simulink model "led_ADC_FW"  (R2024b)
settings: Solver=ode4  StartTime=0.0  StopTime=Inf  FixedStep=Ts  RelTol=1e-3  EnableMultiTasking=on
InitFcn:
  | Ts=1e-4
model workspace (MAT data in the model file):
  encoderResolution = 2000
  hallOffset = '0.5'
  indexOffset = 850
  polePairs = '4'
libraries: c2837xDlib x5, simulink x4, c280xlib x2, c2802xlib x1
(part 1 of 2)
settings Model: ExtModeTrigDuration=8  Creator=matti  LastModifiedBy=Administrator
settings SolverCC: AlgebraicLoopSolver=TrustRegion
settings DataIOCC: LimitDataPoints=on  SaveFormat=Array  SignalLoggingSaveFormat=ModelDataLogs  SaveOutput=off  SaveTime=off  ReturnWorkspaceOutputs=off
settings OptimizationCC: DefaultUnderspecifiedDataType=single  OptimizeBlockIOStorage=off  BufferReuse=off  GlobalBufferReuse=off  ExpressionFolding=off  ExpressionDepthLimit=2147483647  LocalBlockOutputs=off  InitFltsAndDblsToZero=on  NoFixptDivByZeroProtection=on  EfficientFloat2IntCast=on  EfficientMapNaN2IntZero=off  LifeSpan=Inf  MaxStackSize=1024  OptimizeDataStoreBuffers=off  BusAssignmentInplaceUpdate=off  EfficientTunableParamExpr=on
settings DebuggingCC: ReadBeforeWriteMsg=DisableAll  WriteAfterWriteMsg=DisableAll  WriteAfterReadMsg=DisableAll  CheckSSInitialOutputMsg=off  UnderspecifiedInitializationDetection=Classic  MergeDetectMultiDrivingBlocksExec=none  SignalResolutionControl=TryResolveAllWithWarning  SolverPrmCheckMsg=warning  InheritedTsInSrcMsg=none  MultiTaskDSMMsg=none  MultiTaskCondExecSysMsg=none  TasksWithSamePriorityMsg=none  SigSpecEnsureSampleTimeMsg=none  IntegerOverflowMsg=none  ParameterPrecisionLossMsg=none  FcnCallInpInsideContextMsg=warning  UnconnectedInputMsg=warning  UnconnectedOutputMsg=warning  UnconnectedLineMsg=warning  StateNameClashWarn=warning  SFUnexpectedBacktrackingDiag=warning  SFNoUnconditionalDefaultTransitionDiag=warning  SFExecutionAtInitializationDiag=none  IntegerSaturationMsg=none  ArithmeticOperatorsInVariantConditions=warning
settings HardwareCC: ProdBitPerChar=16  ProdBitPerInt=16  ProdBitPerPointer=32  ProdBitPerSizeT=32  ProdBitPerPtrDiffT=32  ProdLargestAtomicInteger=Integer  ProdLargestAtomicFloat=None  ProdWordSize=16  ProdLongLongMode=on  ProdHWDeviceType=Texas Instruments->C2000  TargetBitPerChar=16  TargetBitPerInt=16  TargetBitPerPointer=16  TargetLargestAtomicInteger=Integer  TargetIntDivRoundTo=Zero  TargetEndianess=LittleEndian  TargetWordSize=16  TargetHWDeviceType=TI C2000  HardwareBoardFeatureSet=SoCBlockset
settings ModelReferenceCC: EnableRefExpFcnMdlSchedulingChecks=on  PropagateSignalLabelsOutOfModel=off
settings SFSimCC: SimUseLocalCustomCode=off  MATLABDynamicMemAlloc=off  CustomCodeUndefinedFunction=UseInterfaceOnly
settings RTWCC: Description=Embedded Coder  SystemTargetFile=ert.tlc  HardwareBoard=TI Delfino F28379D LaunchPad  TemplateMakefile=ert_default_tmf  GenerateReport=on  RTWUseLocalCustomCode=off  CustomHeaderCode=#include<stdlib.h>  Toolchain=Texas Instruments Code Composer Studio (C2000)  IncludeHyperlinkInReport=on  LaunchReport=on  CodeProfilingSaveOptions=MetricsOnly  GenerateTraceInfo=on  GenerateTraceReport=on  GenerateTraceReportSl=on  GenerateTraceReportSf=on  GenerateTraceReportEml=on  GPUComputeCapability=3.5
settings CodeAppCC: IgnoreCustomStorageClasses=off  CustomSymbolStrType=$N$R$M  StateflowObjectComments=on  InternalIdentifier=Classic
settings ERTTargetCC: CodeReplacementLibrary=TI C28x  MultiwordLength=2048  SupportContinuousTime=on  ExtModeTransport=4  ExtModeStaticAlloc=on  ExtModeAutomaticAllocSize=off  ExtModeStaticAllocSize=10000  ExtModeMexFile=ext_xcp  ExtModeIntrfLevel=Level2 - Open  InlinedParameterPlacement=Hierarchical  ConvertIfToSwitch=off  SuppressUnreachableDefaultCases=off  MemSecPackage=tic2000demospkg  MemSecFuncExecute=code_ramfuncs  DynamicArrayContainerType=coder::array
settings ConfigComp: CovMetricSettings=dw  CovSaveCumulativeToWorkspaceVar=on  CovSaveSingleToWorkspaceVar=on  CovExternalEMLEnable=off  CovSFcnEnable=off
settings SimscapeCC: SimscapeNormalizeSystem=off

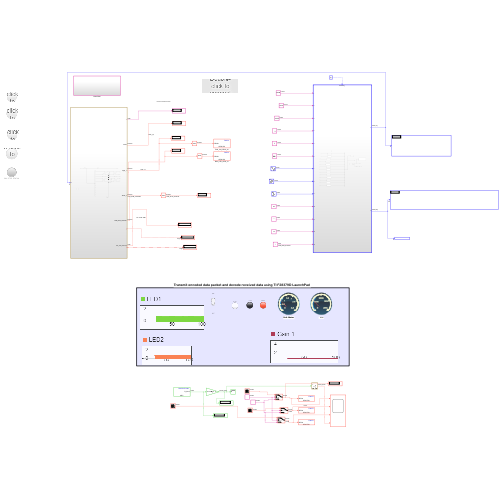
[thumbnail: Simulink's stored preview of the top-level diagram]
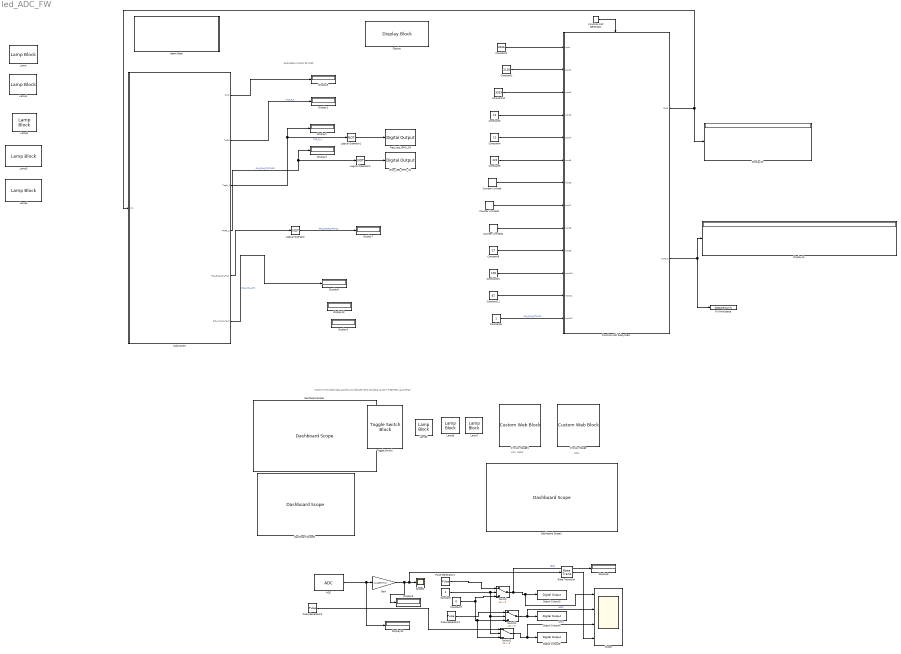
== system led_ADC_FW ==
  note: SHAILESH KUMAR SR MGR
  note: Votl- Meter
  note: Transmit encoded data packet and decode received data using TI F28379D LaunchPad
  note: RPM
  ADC : c2802xlib/ADC  blkParamProc=C2000_Type4  ADCModule=D  samplingMode=Single sample mode  ADCResolution=12-bit (Single-ended input)  useSOC1=SOC0  useSOC2=SOC0_SOC1  SOCAcquisitionWindow=15  SOCTriggerSource=Software  SOCInterruptTrigger=No ADCINT  Ts=0.001  dType=uint16  postInterrupt=off  interruptSel=ADCINT1  ADCINTContinuous=on  endma=off  chdma=1  conv1=ADCINA0  conv2=ADCINA0 and ADCINB0  conv1_Type4=ADCIN14  conv2_Type4=ADCIN0 and ADCIN1
      settings: LibrarySourceBlock=c2837xDlib/ADC
  Blue_LED_GPIO_31 : c2837xDlib/Digital Output  GPIO_Number=GPIO24~GPIO31  GPIO_Bit0=off  GPIO_BIT0_Toggle=off  GPIO_Bit1=off  GPIO_BIT1_Toggle=off  GPIO_Bit2=off  GPIO_BIT2_Toggle=off  GPIO_Bit3=off  GPIO_BIT3_Toggle=off  GPIO_Bit4=off  GPIO_BIT4_Toggle=off  GPIO_Bit5=off  GPIO_BIT5_Toggle=off  GPIO_Bit6=off  GPIO_BIT6_Toggle=off  GPIO_Bit7=on  GPIO_BIT7_Toggle=off
  Circular Gauge : CustomWebBlock  LabelPosition=Hide  ShowInitialText=on  Configuration="{\"components\":[{\"name\":\"CircularScaleComponent\",\"settings\":{\"bounds\":{\"max\":4096,\"min\":0,\"tickInterval\":\"auto\"},\"direction\":\"cw\",\"flipLimits\":0,\"innerRadius\":0.75,\"internalTickHeightScaleFactor\":1,\"labelColor\":[255,255,200],\"labelFont\":{\"font\":\"Arial\",\"fontSize\":12},\"labelRadius\":0.528,\"labelTransparency\":1,\"minorTickHeightScaleFactor\":0.2,\"needleImage\":{\"size\":[200,50],\"src\":\"data:image\\/svg+xml;base64,PD94bWwgdmVyc2lvbj0iMS4wIiBlbmNvZGluZz0idXRmLTgiPz4KPCEtLSBHZW5lcmF0b3I6IEFkb2JlIElsbHVzdHJhdG9yIDI0LjEuMiwgU1ZHIEV4cG9ydCBQbHVnLUluIC4gU1ZHIFZlcnNpb246IDYuMDAgQnVpbGQgMCkgIC0tPgo8c3ZnIHZlcnNpb249IjEuMSIgaWQ9IkxheWVyXzEiIHhtbG5zPSJodHRwOi8vd3d3LnczLm9yZy8yMDAwL3N2ZyIgeG1sbnM6eGxpbms9Imh0dHA6Ly93d3cudzMub3JnLzE5OTkveGxpbmsiIHg9IjBweCIgeT0iMHB4IgoJIHZpZXdCb3g9IjAgMCAyMDAgNTAiIHN0eWxlPSJlbmFibGUtYmFja2dyb3VuZDpuZXcgMCAwIDIwMCA1MDsiIHhtbDpzcGFjZT0icHJlc2VydmUiPgo8c3R5bGUgdHlwZT0idGV4dC9jc3MiPgoJLnN0MHtmaWxsOiNFQzIxMjc7fQo8L3N0eWxlPgo8cGF0aCBjbGFzcz0ic3QwIiBkPSJNMTYyLjgsMTMuN0MxNjksNC40LDE4MS43LDEuOSwxOTEsOC4xczExLjgsMTguOSw1LjYsMjguMnMtMTguOSwxMS44LTI4LjIsNS42bDAsMAoJQzE1OS4xLDM1LjYsMTU2LjYsMjMsMTYyLjgsMTMuN0wxNjIuOCwxMy43eiBNMTY1LjgsMTUuOGMtNS4xLDcuNi0zLjEsMTcuOSw0LjYsMjNjNy42LDUuMSwxNy45LDMuMSwyMy00LjYKCWM1LjEtNy42LDMuMS0xNy45LTQuNi0yM2wwLDBDMTgxLjIsNi4yLDE3MC45LDguMiwxNjUuOCwxNS44eiIvPgo8cGF0aCBjbGFzcz0ic3QwIiBkPSJNMC40LDI1Ljl2LTMuM2wxNTktMi41Yy0wLjcsMi42LTAuNyw1LjIsMCw3LjhMMC40LDI1Ljl6Ii8+CjxjaXJjbGUgY2xhc3M9InN0MCIgY3g9IjE3OS42IiBjeT0iMjQiIHI9IjAuNyIvPgo8L3N2Zz4K\"},\"needleOffset\":[0.18464878250906522,0],\"needleOrientation\":-45,\"needleRotation\":180,\"needleSize\":{\"height\":0.11741692305346914,\"width\":0.46108337545091255},\"outerRadius\":0.9,\"position\":[0.05,0.05,0.9,0.9],\"referencePoint\":\"auto\",\"scaleAngle\":270,\"scaleAngleOffset\":135,\"scaleColors\":[],\"scaleColorsSize\":0.2,\"scaleDirection\":\"CW\",\"scalePosition\":[0,0,1,1],\"showLabels\":1,\"showMinorTicks\":1,\"showSpanLine\":1,\"showTicks\":1,\"tickColor\":[252,252,197],\"tickTransparency\":1,\"valueBarColor\":[0,114,189],\"valueBarPosition\":[0,0,1,1],\"valueBarSize\":0.2,\"valueBarTransparency\":1}},{\"name\":\"BackgroundImageComponent\",\"settings\":{\"image\":{\"size\":[500,500],\"src\":\"data:image\\/svg+xml;base64,PD94bWwgdmVyc2lvbj0iMS4wIiBlbmNvZGluZz0iVVRGLTgiIHN0YW5kYWxvbmU9Im5vIj8+CjxzdmcKICAgeG1sbnM6ZGM9Imh0dHA6Ly9wdXJsLm9yZy9kYy9lbGVtZW50cy8xLjEvIgogICB4bWxuczpjYz0iaHR0cDovL2NyZWF0aXZlY29tbW9ucy5vcmcvbnMjIgogICB4bWxuczpyZGY9Imh0dHA6Ly93d3cudzMub3JnLzE5OTkvMDIvMjItcmRmLXN5bnRheC1ucyMiCiAgIHhtbG5zOnN2Zz0iaHR0cDovL3d3dy53My5vcmcvMjAwMC9zdmciCiAgIHhtbG5zPSJodHRwOi8vd3d3LnczLm9yZy8yMDAwL3N2ZyIKICAgeG1sbnM6 ...(+9964 chars)\"},\"position\":[0,0,1,1],\"scaleMode\":\"0\"}},{\"name\":\"ForegroundImageComponent\",\"settings\":{\"image\":{\"size\":[0,0],\"src\":\"default\",\"srcOrientation\":[]},\"isForeground\":1,\"position\":[0,0,1,1],\"scaleMode\":\"0\"}}],\"settings\":{\"BindingType\":\"signal\",\"aspectRatio\":1.032258064516129,\"backgroundColor\":[0,0,0,\"1\"],\"backgroundOffset\":1,\"backgroundOpacity\":1,\"direction\":\"cw\",\"fixedAspectRatio\":\"on\",\"flipLimits\":0,\"orientation\":\"horizontal\",\"showBackgroundColor\":false,\"value\":0,\"version\":\"R2023a\"},\"type\":\"CircularGauge\"}"
  Circular Gauge1 : CustomWebBlock  LabelPosition=Hide  ShowInitialText=on  Configuration="{\"components\":[{\"name\":\"CircularScaleComponent\",\"settings\":{\"bounds\":{\"max\":3.3,\"min\":0,\"tickInterval\":\"auto\"},\"direction\":\"cw\",\"flipLimits\":0,\"innerRadius\":0.75,\"internalTickHeightScaleFactor\":1,\"labelColor\":[255,255,200],\"labelFont\":{\"font\":\"Arial\",\"fontSize\":12},\"labelRadius\":0.528,\"labelTransparency\":1,\"minorTickHeightScaleFactor\":0.2,\"needleImage\":{\"size\":[200,50],\"src\":\"data:image\\/svg+xml;base64,PD94bWwgdmVyc2lvbj0iMS4wIiBlbmNvZGluZz0idXRmLTgiPz4KPCEtLSBHZW5lcmF0b3I6IEFkb2JlIElsbHVzdHJhdG9yIDI0LjEuMiwgU1ZHIEV4cG9ydCBQbHVnLUluIC4gU1ZHIFZlcnNpb246IDYuMDAgQnVpbGQgMCkgIC0tPgo8c3ZnIHZlcnNpb249IjEuMSIgaWQ9IkxheWVyXzEiIHhtbG5zPSJodHRwOi8vd3d3LnczLm9yZy8yMDAwL3N2ZyIgeG1sbnM6eGxpbms9Imh0dHA6Ly93d3cudzMub3JnLzE5OTkveGxpbmsiIHg9IjBweCIgeT0iMHB4IgoJIHZpZXdCb3g9IjAgMCAyMDAgNTAiIHN0eWxlPSJlbmFibGUtYmFja2dyb3VuZDpuZXcgMCAwIDIwMCA1MDsiIHhtbDpzcGFjZT0icHJlc2VydmUiPgo8c3R5bGUgdHlwZT0idGV4dC9jc3MiPgoJLnN0MHtmaWxsOiNFQzIxMjc7fQo8L3N0eWxlPgo8cGF0aCBjbGFzcz0ic3QwIiBkPSJNMTYyLjgsMTMuN0MxNjksNC40LDE4MS43LDEuOSwxOTEsOC4xczExLjgsMTguOSw1LjYsMjguMnMtMTguOSwxMS44LTI4LjIsNS42bDAsMAoJQzE1OS4xLDM1LjYsMTU2LjYsMjMsMTYyLjgsMTMuN0wxNjIuOCwxMy43eiBNMTY1LjgsMTUuOGMtNS4xLDcuNi0zLjEsMTcuOSw0LjYsMjNjNy42LDUuMSwxNy45LDMuMSwyMy00LjYKCWM1LjEtNy42LDMuMS0xNy45LTQuNi0yM2wwLDBDMTgxLjIsNi4yLDE3MC45LDguMiwxNjUuOCwxNS44eiIvPgo8cGF0aCBjbGFzcz0ic3QwIiBkPSJNMC40LDI1Ljl2LTMuM2wxNTktMi41Yy0wLjcsMi42LTAuNyw1LjIsMCw3LjhMMC40LDI1Ljl6Ii8+CjxjaXJjbGUgY2xhc3M9InN0MCIgY3g9IjE3OS42IiBjeT0iMjQiIHI9IjAuNyIvPgo8L3N2Zz4K\"},\"needleOffset\":[0.18464878250906522,0],\"needleOrientation\":-45,\"needleRotation\":180,\"needleSize\":{\"height\":0.11741692305346914,\"width\":0.46108337545091255},\"outerRadius\":0.9,\"position\":[0.05,0.05,0.9,0.9],\"referencePoint\":\"auto\",\"scaleAngle\":270,\"scaleAngleOffset\":135,\"scaleColors\":[],\"scaleColorsSize\":0.2,\"scaleDirection\":\"CW\",\"scalePosition\":[0,0,1,1],\"showLabels\":1,\"showMinorTicks\":1,\"showSpanLine\":1,\"showTicks\":1,\"tickColor\":[252,252,197],\"tickTransparency\":1,\"valueBarColor\":[0,114,189],\"valueBarPosition\":[0,0,1,1],\"valueBarSize\":0.2,\"valueBarTransparency\":1}},{\"name\":\"BackgroundImageComponent\",\"settings\":{\"image\":{\"size\":[500,500],\"src\":\"data:image\\/svg+xml;base64,PD94bWwgdmVyc2lvbj0iMS4wIiBlbmNvZGluZz0iVVRGLTgiIHN0YW5kYWxvbmU9Im5vIj8+CjxzdmcKICAgeG1sbnM6ZGM9Imh0dHA6Ly9wdXJsLm9yZy9kYy9lbGVtZW50cy8xLjEvIgogICB4bWxuczpjYz0iaHR0cDovL2NyZWF0aXZlY29tbW9ucy5vcmcvbnMjIgogICB4bWxuczpyZGY9Imh0dHA6Ly93d3cudzMub3JnLzE5OTkvMDIvMjItcmRmLXN5bnRheC1ucyMiCiAgIHhtbG5zOnN2Zz0iaHR0cDovL3d3dy53My5vcmcvMjAwMC9zdmciCiAgIHhtbG5zPSJodHRwOi8vd3d3LnczLm9yZy8yMDAwL3N2ZyIKICAgeG1sbnM6 ...(+9964 chars)\"},\"position\":[0,0,1,1],\"scaleMode\":\"0\"}},{\"name\":\"ForegroundImageComponent\",\"settings\":{\"image\":{\"size\":[0,0],\"src\":\"default\",\"srcOrientation\":[]},\"isForeground\":1,\"position\":[0,0,1,1],\"scaleMode\":\"0\"}}],\"settings\":{\"BindingType\":\"signal\",\"aspectRatio\":1.032258064516129,\"backgroundColor\":[0,0,0,\"1\"],\"backgroundOffset\":1,\"backgroundOpacity\":1,\"direction\":\"cw\",\"fixedAspectRatio\":\"on\",\"flipLimits\":0,\"orientation\":\"horizontal\",\"showBackgroundColor\":false,\"value\":0,\"version\":\"R2023a\"},\"type\":\"CircularGauge\"}"
  Constant : Constant
  Constant1 : Constant  Value=2130  OutDataTypeStr=uint16
  Constant10 : Constant  Value=100  OutDataTypeStr=uint16
  Constant11 : Constant  Value=67  OutDataTypeStr=uint16
  Constant12 : Constant  Value=3333  OutDataTypeStr=uint16
  Constant2 : Constant  Value=3046  OutDataTypeStr=uint16
  Constant3 : Constant  Value=12  OutDataTypeStr=uint16
  Constant4 : Constant  Value=11  OutDataTypeStr=uint16
  Constant5 : Constant  Value=222  OutDataTypeStr=uint16
  Constant6 : Constant  OutDataTypeStr=uint8
  Constant7 : Constant  Value=0
  Constant9 : Constant  Value=27  OutDataTypeStr=uint16
  Counter Limited : simulink/Sources/Counter Limited  uplimit=999  tsamp=-1
  Counter Limited1 : simulink/Sources/Counter Limited  uplimit=999  tsamp=-1
  Counter Limited2 : simulink/Sources/Counter Limited  uplimit=999  tsamp=-1
  Dashboard Scope : DashboardScope  Ymin=-1  Ymax=2  NormalizeYAxis=on  TicksPosition=Inside
  Dashboard Scope1 : DashboardScope  Ymin=.5  Ymax=4  UpdateMode=Scroll  NormalizeYAxis=on  TicksPosition=Inside
  Dashboard Scope2 : DashboardScope  Ymin=-1  Ymax=2  UpdateMode=Scroll  NormalizeYAxis=on  TicksPosition=Inside
  Digital Output3 : c2837xDlib/Digital Output  GPIO_Number=GPIO0~GPIO7  GPIO_Bit0=on  GPIO_BIT0_Toggle=off  GPIO_Bit1=off  GPIO_BIT1_Toggle=off  GPIO_Bit2=off  GPIO_BIT2_Toggle=off  GPIO_Bit3=off  GPIO_BIT3_Toggle=off  GPIO_Bit4=off  GPIO_BIT4_Toggle=off  GPIO_Bit5=off  GPIO_BIT5_Toggle=off  GPIO_Bit6=off  GPIO_BIT6_Toggle=off  GPIO_Bit7=off  GPIO_BIT7_Toggle=off
  Digital Output4 : c2837xDlib/Digital Output  GPIO_Number=GPIO0~GPIO7  GPIO_Bit0=off  GPIO_BIT0_Toggle=off  GPIO_Bit1=on  GPIO_BIT1_Toggle=off  GPIO_Bit2=off  GPIO_BIT2_Toggle=off  GPIO_Bit3=off  GPIO_BIT3_Toggle=off  GPIO_Bit4=off  GPIO_BIT4_Toggle=off  GPIO_Bit5=off  GPIO_BIT5_Toggle=off  GPIO_Bit6=off  GPIO_BIT6_Toggle=off  GPIO_Bit7=off  GPIO_BIT7_Toggle=off
  Digital Output5 : c2837xDlib/Digital Output  GPIO_Number=GPIO0~GPIO7  GPIO_Bit0=off  GPIO_BIT0_Toggle=off  GPIO_Bit1=off  GPIO_BIT1_Toggle=off  GPIO_Bit2=on  GPIO_BIT2_Toggle=off  GPIO_Bit3=off  GPIO_BIT3_Toggle=off  GPIO_Bit4=off  GPIO_BIT4_Toggle=off  GPIO_Bit5=off  GPIO_BIT5_Toggle=off  GPIO_Bit6=off  GPIO_BIT6_Toggle=off  GPIO_Bit7=off  GPIO_BIT7_Toggle=off
  Display : DisplayBlock  Transparency=1
  Display{1..10,13..15} (13 alike) : Display
  Function-Call Generator : simulink/Ports & Subsystems/Function-Call Generator  sample_time=0.1  numberOfIterations=1  DisallowWideOutput=off
  Function-Call Subsystem : Subsystem  TreatAsAtomicUnit=on
  Gain : Gain  Gain=(1/4095)*3.3
  Heart-Beat : Subsystem
  Lamp{,1..2,5..7} (6 alike) : LampBlock
  Lamp3 : LampBlock  LabelPosition=Bottom
  Lamp4 : LampBlock  LabelPosition=Bottom
  Logical Operator : Logic  Operator=NOT  AllPortsSameDT=off  OutDataTypeStr=boolean
  Logical Operator1 : Logic  Operator=NOT  AllPortsSameDT=off  OutDataTypeStr=boolean
  Logical Operator2 : Logic  Operator=NOT  AllPortsSameDT=off  OutDataTypeStr=boolean
  Pulse Generator1 : DiscretePulseGenerator  PulseType=Time based  Amplitude=0.5  Period=500e-3  PulseWidth=50  SampleTime=0.1
  Pulse Generator2 : DiscretePulseGenerator  PulseType=Time based  Amplitude=0.5  Period=1  PulseWidth=50  SampleTime=0.1
  Pulse Generator3 : DiscretePulseGenerator  PulseType=Time based  Amplitude=0.5  PulseWidth=50  SampleTime=0.1
  Rate Transition : RateTransition
  Red_Led_GPIO_34 : c2837xDlib/Digital Output  GPIO_Number=GPIO32~GPIO39  GPIO_Bit0=off  GPIO_BIT0_Toggle=off  GPIO_Bit1=off  GPIO_BIT1_Toggle=off  GPIO_Bit2=on  GPIO_BIT2_Toggle=off  GPIO_Bit3=off  GPIO_BIT3_Toggle=off  GPIO_Bit4=off  GPIO_BIT4_Toggle=off  GPIO_Bit5=off  GPIO_BIT5_Toggle=off  GPIO_Bit6=off  GPIO_BIT6_Toggle=off  GPIO_Bit7=off  GPIO_BIT7_Toggle=off
  Scope : Scope  NumInputPorts=4
  Scope1 : Scope
  Subsystem : Subsystem
  Switch : Switch  Criteria=u2 > Threshold  SaturateOnIntegerOverflow=off  InputSameDT=off
  Switch1 : Switch  Criteria=u2 > Threshold  SaturateOnIntegerOverflow=off  InputSameDT=off
  Switch2 : Switch  Criteria=u2 > Threshold  SaturateOnIntegerOverflow=off  InputSameDT=off
  To Workspace : ToWorkspace  VariableName=datatransmit  SampleTime=-1
      settings: Save2DSignal=2-D array (concatenate along first dimension)
  Toggle Switch : ToggleSwitchBlock  LabelPosition=Hide
      settings: Values={{'Off', 'On'}, [0 1]}
  wires:
  Subsystem/1(Out1) -> Display5/1
  Subsystem/3(Tag9_1) -> Display2/1, Logical Operator1/1  "TAG_9_1"
  Subsystem/6(DC_Link_Current) -> Display6/1  "DC_LINK_AMP"
  Subsystem/2(TAG9) -> Display1/1  "TAG_9_0"
  Logical Operator/1 -> Display7/1  "FAN_STOP_STATUS"
  Function-Call Generator/1 -> Function-Call Subsystem/Trigger
  Function-Call Subsystem/1(Out2) -> Subsystem/1(In1), Display15/1
  Constant2/1 -> Function-Call Subsystem/1(Input)
  Constant1/1 -> Function-Call Subsystem/2(Input1)
  Constant12/1 -> Function-Call Subsystem/3(Input2)
  Constant3/1 -> Function-Call Subsystem/4(Input3)
  Constant4/1 -> Function-Call Subsystem/5(Input4)
  Constant5/1 -> Function-Call Subsystem/6(Input5)
  Counter Limited/1 -> Function-Call Subsystem/7(Input6)
  Counter Limited1/1 -> Function-Call Subsystem/8(Input7)
  Counter Limited2/1 -> Function-Call Subsystem/9(Input8)
  Constant9/1 -> Function-Call Subsystem/10(Input9)
  Constant10/1 -> Function-Call Subsystem/11(Input10)
  Constant11/1 -> Function-Call Subsystem/12(Input11)
  Constant6/1 -> Function-Call Subsystem/13(Input12)  "FAN_RUN_STATUS"
  Function-Call Subsystem/2(Output) -> To Workspace/1, Display14/1
  Logical Operator1/1 -> Red_Led_GPIO_34/1
  Logical Operator2/1 -> Blue_LED_GPIO_31/1
  Subsystem/4(TAG9_2) -> Display3/1, Logical Operator2/1  "FAN_RUN_STATUSS"
  Subsystem/5(FAN_RUN_STATUS) -> Logical Operator/1
  ? -> Display13/1
  ? -> Display4/1
  Pulse Generator3/1 -> Switch2/1
  Rate Transition/1 -> Scope/4
  Pulse Generator1/1 -> Switch/1
  Pulse Generator2/1 -> Switch1/1
  ADC/1 -> Display10/1, Gain/1
  Switch1/1 -> Scope/2, Digital Output4/1  "LED2"
  Constant/1 -> Switch2/2, Switch1/2, Switch/2
  Gain/1 -> Display9/1, Rate Transition/1, Scope1/1
  Constant7/1 -> Switch/3, Switch2/3, Switch1/3
  Switch/1 -> Display8/1, Scope/1, Digital Output3/1  "LED1"
  Switch2/1 -> Scope/3, Digital Output5/1  "LED3"

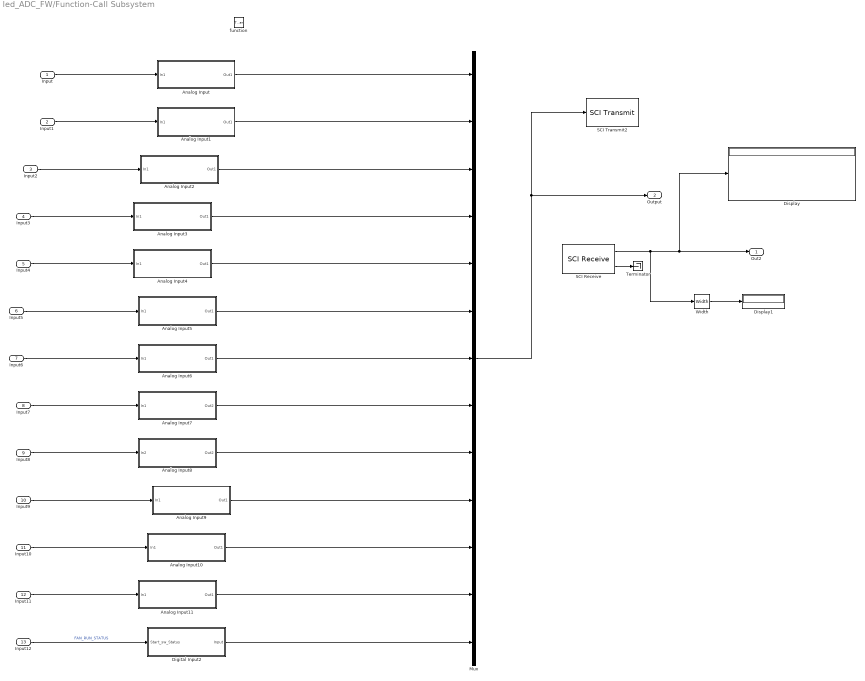
== system led_ADC_FW/Function-Call Subsystem ==
  Input : Inport
  Input1 : Inport  Port=2
  Input2 : Inport  Port=3
  Input3 : Inport  Port=4
  Input4 : Inport  Port=5
  Input5 : Inport  Port=6
  Input6 : Inport  Port=7
  Input7 : Inport  Port=8
  Input8 : Inport  Port=9
  Input9 : Inport  Port=10
  Input10 : Inport  Port=11
  Input11 : Inport  Port=12
  Input12 : Inport  Port=13
  function : TriggerPort  TriggerType=function-call  VariantControl=(inherit)
  Analog Input : Subsystem
  Analog Input1 : Subsystem
  Analog Input10 : Subsystem
  Analog Input11 : Subsystem
  Analog Input2 : Subsystem
  Analog Input3 : Subsystem
  Analog Input4 : Subsystem
  Analog Input5 : Subsystem
  Analog Input6 : Subsystem
  Analog Input7 : Subsystem
  Analog Input8 : Subsystem
  Analog Input9 : Subsystem
  Digital Input2 : Subsystem
  Display : Display
  Display1 : Display
  Mux : Mux  Inputs=13
  SCI Receive : c280xlib/SCI Receive  Priority=2  sciModule=B  dataHead='S'  headerCheckMaxCount=16  dataTail='E'  dataType=uint8  dataLenOptions=Length via dialog  dataDim=11  maxDataLength=1  initValue=0  errOption=Output the last received value  errValue=0  sampleTime=-1  blockingMode=off  timeOut=inf  outputStatus=on
      settings: LibrarySourceBlock=c2837xDlib/SCI Receive
  SCI Transmit2 : c280xlib/SCI Transmit  sciModule=B  dataHead='S'  dataTail='E'  frameSize=[1 49]  blockingMode=on  outputStatus=off
      settings: LibrarySourceBlock=c2837xDlib/SCI Transmit
  Terminator : Terminator
  Width : Width  DataType=uint8
  Out2 : Outport
  Output : Outport  Port=2
  wires:
  SCI Receive/1 -> Width/1, Display/1, Out2/1
  SCI Receive/2 -> Terminator/1
  Digital Input2/1(Input) -> Mux/13
  Analog Input/1(Out1) -> Mux/1
  Input/1 -> Analog Input/1(In1)
  Input12/1 -> Digital Input2/1(Start_sw_Status)  "FAN_RUN_STATUS"
  Mux/1 -> SCI Transmit2/1, Output/1
  Width/1 -> Display1/1
  Input1/1 -> Analog Input1/1(In1)
  Analog Input1/1(Out1) -> Mux/2
  Input2/1 -> Analog Input2/1(In1)
  Analog Input2/1(Out1) -> Mux/3
  Input3/1 -> Analog Input3/1(In1)
  Analog Input3/1(Out1) -> Mux/4
  Input4/1 -> Analog Input4/1(In1)
  Analog Input4/1(Out1) -> Mux/5
  Input5/1 -> Analog Input5/1(In1)
  Analog Input5/1(Out1) -> Mux/6
  Input6/1 -> Analog Input6/1(In1)
  Analog Input6/1(Out1) -> Mux/7
  Input7/1 -> Analog Input7/1(In1)
  Analog Input7/1(Out2) -> Mux/8
  Input8/1 -> Analog Input8/1(In2)
  Analog Input8/1(Out2) -> Mux/9
  Input9/1 -> Analog Input9/1(In1)
  Analog Input9/1(Out1) -> Mux/10
  Input10/1 -> Analog Input10/1(In1)
  Analog Input10/1(Out1) -> Mux/11
  Input11/1 -> Analog Input11/1(In1)
  Analog Input11/1(Out1) -> Mux/12

== system led_ADC_FW/Heart-Beat ==

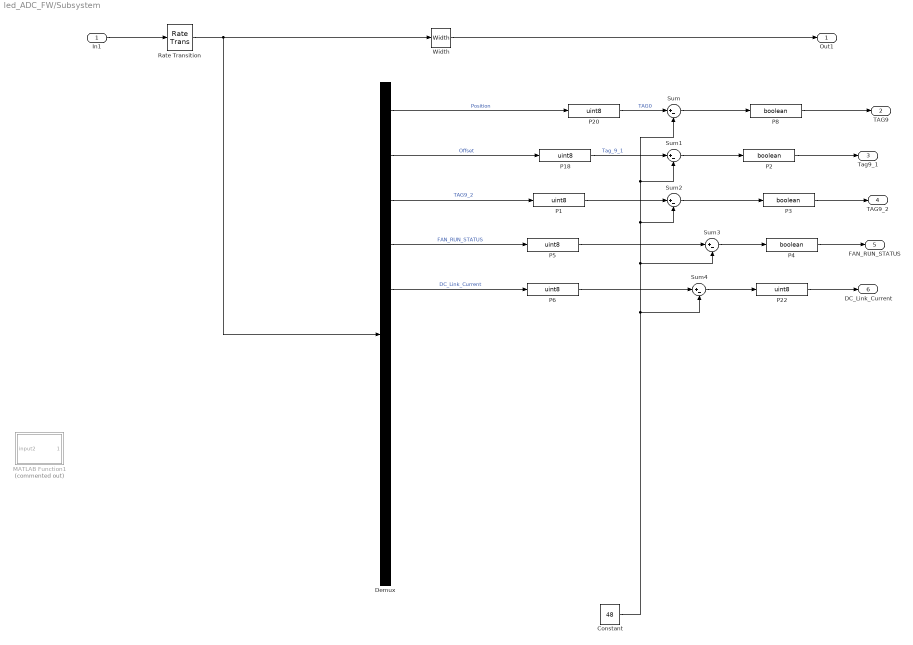
== system led_ADC_FW/Subsystem ==
  In1 : Inport
  Constant : Constant  Value=48  OutDataTypeStr=uint8
  Demux : Demux  Outputs=11
  MATLAB Function1 : MATLAB Function  Commented=on  TreatAsAtomicUnit=on
  P{1,5..6,18,20,22} (6 alike) : DataTypeConversion  OutDataTypeStr=uint8  SaturateOnIntegerOverflow=off  RndMeth=Floor
  P{2..4,8} (4 alike) : DataTypeConversion  OutDataTypeStr=boolean  SaturateOnIntegerOverflow=off  RndMeth=Floor
  Rate Transition : RateTransition
  Sum{,1..4} (5 alike) : Sum  Inputs=|+-
  Width : Width  DataType=uint8
  Out1 : Outport
  TAG9 : Outport  Port=2
  Tag9_1 : Outport  Port=3
  TAG9_2 : Outport  Port=4
  FAN_RUN_STATUS : Outport  Port=5
  DC_Link_Current : Outport  Port=6
  wires:
  Demux/1 -> P20/1  "Position"
  P1/1 -> Sum2/1
  P3/1 -> TAG9_2/1
  Sum1/1 -> P2/1
  P2/1 -> Tag9_1/1
  Sum/1 -> P8/1
  P18/1 -> Sum1/1  "Tag_9_1"
  P6/1 -> Sum4/1
  Demux/5 -> P6/1  "DC_Link_Current"
  P4/1 -> FAN_RUN_STATUS/1
  Demux/4 -> P5/1  "FAN_RUN_STATUS"
  P5/1 -> Sum3/1
  Sum3/1 -> P4/1
  Demux/3 -> P1/1  "TAG9_2"
  Sum4/1 -> P22/1
  Demux/2 -> P18/1  "Offset"
  Sum2/1 -> P3/1
  In1/1 -> Rate Transition/1
  Width/1 -> Out1/1
  P20/1 -> Sum/1  "TAG0"
  Rate Transition/1 -> Demux/1, Width/1
  P8/1 -> TAG9/1
  P22/1 -> DC_Link_Current/1
  Constant/1 -> Sum4/2, Sum3/2, Sum2/2, Sum1/2, Sum/2

== system led_ADC_FW/Function-Call Subsystem/Analog Input ==
  In1 : Inport
  Subsystem : Subsystem
  Out1 : Outport
  wires:
  Subsystem/1(Out1) -> Out1/1
  In1/1 -> Subsystem/1(In1)

== system led_ADC_FW/Function-Call Subsystem/Analog Input1 ==
  In1 : Inport
  Subsystem : Subsystem
  Out1 : Outport
  wires:
  Subsystem/1(Out1) -> Out1/1
  In1/1 -> Subsystem/1(In1)

== system led_ADC_FW/Function-Call Subsystem/Analog Input10 ==
  In1 : Inport
  Subsystem : Subsystem
  Out1 : Outport
  wires:
  Subsystem/1(Out1) -> Out1/1
  In1/1 -> Subsystem/1(In1)

== system led_ADC_FW/Function-Call Subsystem/Analog Input11 ==
  In1 : Inport
  Subsystem : Subsystem
  Out1 : Outport
  wires:
  Subsystem/1(Out1) -> Out1/1
  In1/1 -> Subsystem/1(In1)

== system led_ADC_FW/Function-Call Subsystem/Analog Input2 ==
  In1 : Inport
  Subsystem : Subsystem
  Out1 : Outport
  wires:
  Subsystem/1(Out1) -> Out1/1
  In1/1 -> Subsystem/1(In1)

== system led_ADC_FW/Function-Call Subsystem/Analog Input3 ==
  In1 : Inport
  Subsystem : Subsystem
  Out1 : Outport
  wires:
  Subsystem/1(Out1) -> Out1/1
  In1/1 -> Subsystem/1(In1)

== system led_ADC_FW/Function-Call Subsystem/Analog Input4 ==
  In1 : Inport
  Subsystem : Subsystem
  Out1 : Outport
  wires:
  Subsystem/1(Out1) -> Out1/1
  In1/1 -> Subsystem/1(In1)

== system led_ADC_FW/Function-Call Subsystem/Analog Input5 ==
  In1 : Inport
  Subsystem : Subsystem
  Out1 : Outport
  wires:
  Subsystem/1(Out1) -> Out1/1
  In1/1 -> Subsystem/1(In1)

== system led_ADC_FW/Function-Call Subsystem/Analog Input6 ==
  In1 : Inport
  Subsystem : Subsystem
  Out1 : Outport
  wires:
  Subsystem/1(Out1) -> Out1/1
  In1/1 -> Subsystem/1(In1)

== system led_ADC_FW/Function-Call Subsystem/Analog Input7 ==
  In1 : Inport
  Subsystem : Subsystem
  Out2 : Outport
  wires:
  Subsystem/1(Out1) -> Out2/1
  In1/1 -> Subsystem/1(In1)

== system led_ADC_FW/Function-Call Subsystem/Analog Input8 ==
  In2 : Inport
  Subsystem1 : Subsystem
  Out2 : Outport
  wires:
  Subsystem1/1(Out1) -> Out2/1
  In2/1 -> Subsystem1/1(In1)

== system led_ADC_FW/Function-Call Subsystem/Analog Input9 ==
  In1 : Inport
  Subsystem : Subsystem
  Out1 : Outport
  wires:
  Subsystem/1(Out1) -> Out1/1
  In1/1 -> Subsystem/1(In1)

== system led_ADC_FW/Function-Call Subsystem/Digital Input2 ==
  Start_sw_Status : Inport
  Ground10 : Constant  Value=48  OutDataTypeStr=int16
  Saturation1 : Saturate  UpperLimit=1  LowerLimit=0  OutDataTypeStr=double
  Sum4 : Sum  OutDataTypeStr=uint8
  Input : Outport
  wires:
  Saturation1/1 -> Sum4/1
  Start_sw_Status/1 -> Saturation1/1
  Ground10/1 -> Sum4/2
  Sum4/1 -> Input/1

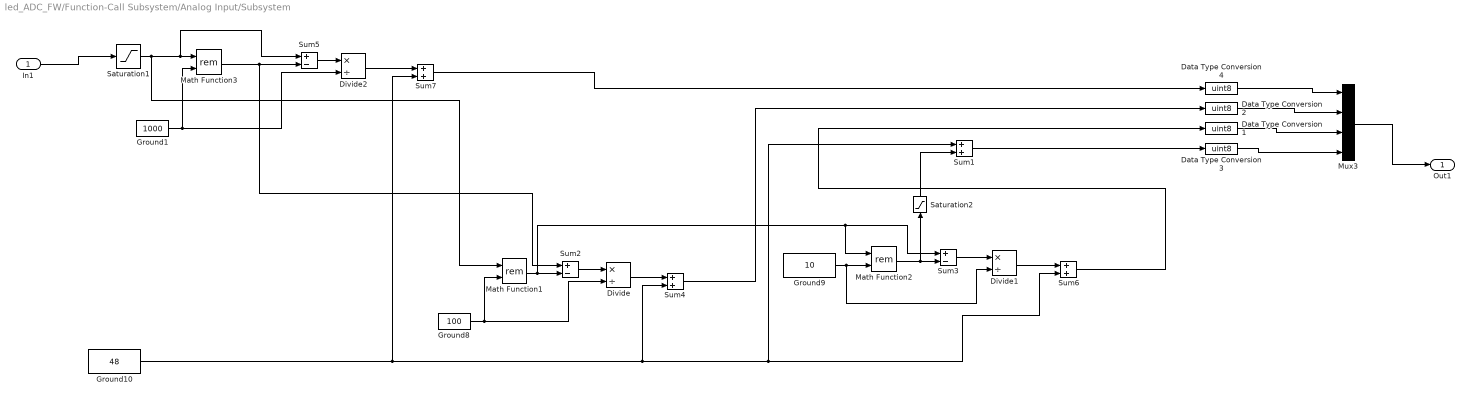
== system led_ADC_FW/Function-Call Subsystem/Analog Input/Subsystem ==
  In1 : Inport
  Data Type Conversion{1..4} (4 alike) : DataTypeConversion  OutDataTypeStr=uint8  SaturateOnIntegerOverflow=off  RndMeth=Floor
  Divide : Product  Inputs=*/  OutDataTypeStr=int16
  Divide1 : Product  Inputs=*/  OutDataTypeStr=int16
  Divide2 : Product  Inputs=*/  OutDataTypeStr=int16
  Ground1 : Constant  Value=1000  OutDataTypeStr=int16
  Ground10 : Constant  Value=48  OutDataTypeStr=int16
  Ground8 : Constant  Value=100  OutDataTypeStr=int16
  Ground9 : Constant  Value=10  OutDataTypeStr=int16
  Math Function1 : Math  Operator=rem  SignedPower=on
  Math Function2 : Math  Operator=rem  SignedPower=on
  Math Function3 : Math  Operator=rem  SignedPower=on
  Mux3 : Mux
  Saturation1 : Saturate  UpperLimit=4096  LowerLimit=0  OutDataTypeStr=int16
  Saturation2 : Saturate  UpperLimit=9  LowerLimit=0
  Sum{1,4,6..7} (4 alike) : Sum  OutDataTypeStr=uint8
  Sum2 : Sum  Inputs=+-  OutDataTypeStr=double
  Sum3 : Sum  Inputs=+-
  Sum5 : Sum  Inputs=+-  OutDataTypeStr=double
  Out1 : Outport
  wires:
  Data Type Conversion2/1 -> Mux3/2
  Sum5/1 -> Divide2/1
  Ground10/1 -> Sum7/2, Sum4/2, Sum6/2, Sum1/1
  Math Function1/1 -> Sum2/2, Math Function2/1, Sum3/1
  Saturation1/1 -> Math Function1/1, Sum5/1, Math Function3/1
  Saturation2/1 -> Sum1/2
  In1/1 -> Saturation1/1
  Divide2/1 -> Sum7/1
  Data Type Conversion1/1 -> Mux3/3
  Sum4/1 -> Data Type Conversion2/1
  Math Function3/1 -> Sum2/1, Sum5/2
  Data Type Conversion4/1 -> Mux3/1
  Sum2/1 -> Divide/1
  Ground9/1 -> Divide1/2, Math Function2/2
  Sum6/1 -> Data Type Conversion1/1
  Ground8/1 -> Divide/2, Math Function1/2
  Ground1/1 -> Divide2/2, Math Function3/2
  Math Function2/1 -> Sum3/2, Saturation2/1
  Data Type Conversion3/1 -> Mux3/4
  Sum1/1 -> Data Type Conversion3/1
  Divide/1 -> Sum4/1
  Divide1/1 -> Sum6/1
  Sum7/1 -> Data Type Conversion4/1
  Sum3/1 -> Divide1/1
  Mux3/1 -> Out1/1

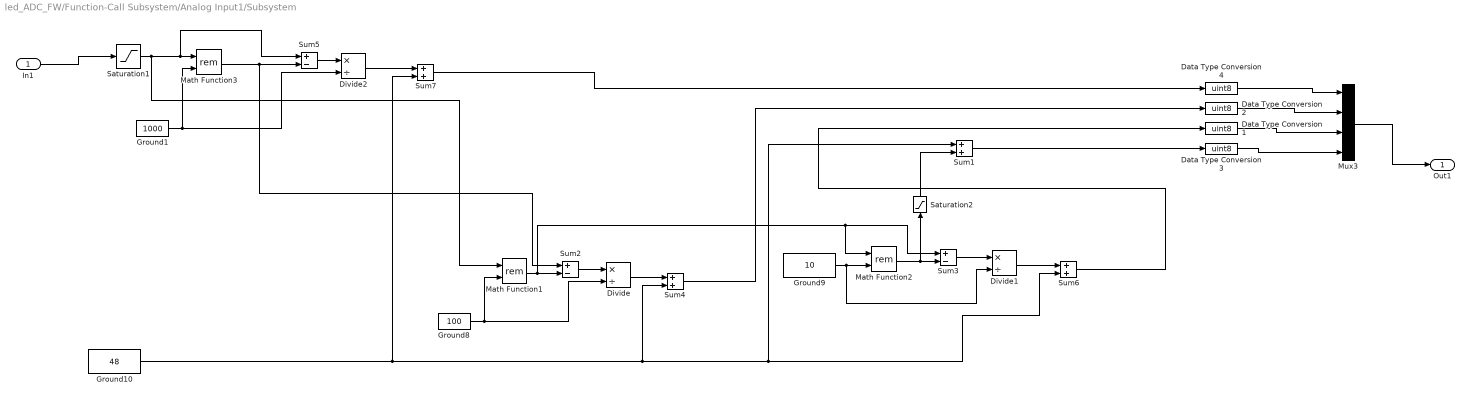
== system led_ADC_FW/Function-Call Subsystem/Analog Input1/Subsystem ==
  In1 : Inport
  Data Type Conversion{1..4} (4 alike) : DataTypeConversion  OutDataTypeStr=uint8  SaturateOnIntegerOverflow=off  RndMeth=Floor
  Divide : Product  Inputs=*/  OutDataTypeStr=int16
  Divide1 : Product  Inputs=*/  OutDataTypeStr=int16
  Divide2 : Product  Inputs=*/  OutDataTypeStr=int16
  Ground1 : Constant  Value=1000  OutDataTypeStr=int16
  Ground10 : Constant  Value=48  OutDataTypeStr=int16
  Ground8 : Constant  Value=100  OutDataTypeStr=int16
  Ground9 : Constant  Value=10  OutDataTypeStr=int16
  Math Function1 : Math  Operator=rem  SignedPower=on
  Math Function2 : Math  Operator=rem  SignedPower=on
  Math Function3 : Math  Operator=rem  SignedPower=on
  Mux3 : Mux
  Saturation1 : Saturate  UpperLimit=4096  LowerLimit=0  OutDataTypeStr=int16
  Saturation2 : Saturate  UpperLimit=9  LowerLimit=0
  Sum{1,4,6..7} (4 alike) : Sum  OutDataTypeStr=uint8
  Sum2 : Sum  Inputs=+-  OutDataTypeStr=double
  Sum3 : Sum  Inputs=+-
  Sum5 : Sum  Inputs=+-  OutDataTypeStr=double
  Out1 : Outport
  wires:
  Data Type Conversion2/1 -> Mux3/2
  Sum5/1 -> Divide2/1
  Ground10/1 -> Sum7/2, Sum4/2, Sum6/2, Sum1/1
  Math Function1/1 -> Sum2/2, Math Function2/1, Sum3/1
  Saturation1/1 -> Math Function1/1, Sum5/1, Math Function3/1
  Saturation2/1 -> Sum1/2
  In1/1 -> Saturation1/1
  Divide2/1 -> Sum7/1
  Data Type Conversion1/1 -> Mux3/3
  Sum4/1 -> Data Type Conversion2/1
  Math Function3/1 -> Sum2/1, Sum5/2
  Data Type Conversion4/1 -> Mux3/1
  Sum2/1 -> Divide/1
  Ground9/1 -> Divide1/2, Math Function2/2
  Sum6/1 -> Data Type Conversion1/1
  Ground8/1 -> Divide/2, Math Function1/2
  Ground1/1 -> Divide2/2, Math Function3/2
  Math Function2/1 -> Sum3/2, Saturation2/1
  Data Type Conversion3/1 -> Mux3/4
  Sum1/1 -> Data Type Conversion3/1
  Divide/1 -> Sum4/1
  Divide1/1 -> Sum6/1
  Sum7/1 -> Data Type Conversion4/1
  Sum3/1 -> Divide1/1
  Mux3/1 -> Out1/1
